simulink model "zadacha_16_02"  (Simulink 7.1)
settings: Solver=ode45  StartTime=0.0  StopTime=100  RelTol=1e-3
settings Model: Creator=Slavi  LastModifiedBy=Slavi

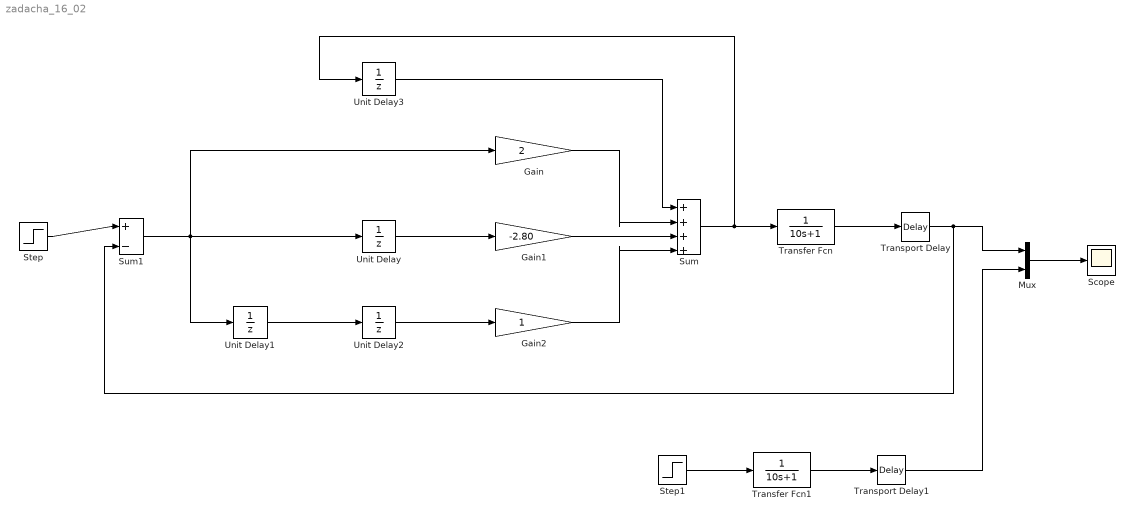
== system zadacha_16_02 ==
  Gain : Gain  Gain=2  ParameterDataType=sfix(16)  ParameterScaling=2^0  OutDataType=sfix(16)  OutScaling=2^0
  Gain1 : Gain  Gain=-2.80  ParameterDataType=sfix(16)  ParameterScaling=2^0  OutDataType=sfix(16)  OutScaling=2^0
  Gain2 : Gain  ParameterDataType=sfix(16)  ParameterScaling=2^0  OutDataType=sfix(16)  OutScaling=2^0
  Mux : Mux  Inputs=2
  Scope : Scope
  Step : Step
  Step1 : Step
  Sum : Sum  Inputs=|++++  OutDataType=sfix(16)  OutScaling=2^0
  Sum1 : Sum  Inputs=|+-  OutDataType=sfix(16)  OutScaling=2^0
  Transfer Fcn : TransferFcn  Denominator=[10 1]
  Transfer Fcn1 : TransferFcn  Denominator=[10 1]
  Transport Delay : TransportDelay  DelayTime=2
  Transport Delay1 : TransportDelay  DelayTime=2
  Unit Delay{,1..3} (4 alike) : UnitDelay
  wires:
  Unit Delay/1 -> Gain1/1
  Unit Delay2/1 -> Gain2/1
  Unit Delay1/1 -> Unit Delay2/1
  Gain/1 -> Sum/2
  Gain1/1 -> Sum/3
  Gain2/1 -> Sum/4
  Sum/1 -> Unit Delay3/1, Transfer Fcn/1
  Unit Delay3/1 -> Sum/1
  Sum1/1 -> Unit Delay/1, Gain/1, Unit Delay1/1
  Mux/1 -> Scope/1
  Step/1 -> Sum1/1
  Transfer Fcn/1 -> Transport Delay/1
  Transport Delay/1 -> Mux/1, Sum1/2
  Step1/1 -> Transfer Fcn1/1
  Transfer Fcn1/1 -> Transport Delay1/1
  Transport Delay1/1 -> Mux/2
